simulink library "ObjSelect_lib"  (R2019b)
settings: Solver=VariableStepAuto  StartTime=0.0  StopTime=10.0  RelTol=1e-3
libraries: $bdroot x1
settings Model: Creator=liuyi  LastModifiedBy=86156
settings DataIOCC: ReturnWorkspaceOutputs=off
settings DebuggingCC: ArithmeticOperatorsInVariantConditions=warning
settings SFSimCC: SimUseLocalCustomCode=off  CustomCodeUndefinedFunction=UseInterfaceOnly
settings RTWCC: RTWUseLocalCustomCode=off
settings CodeAppCC: StateflowObjectComments=on

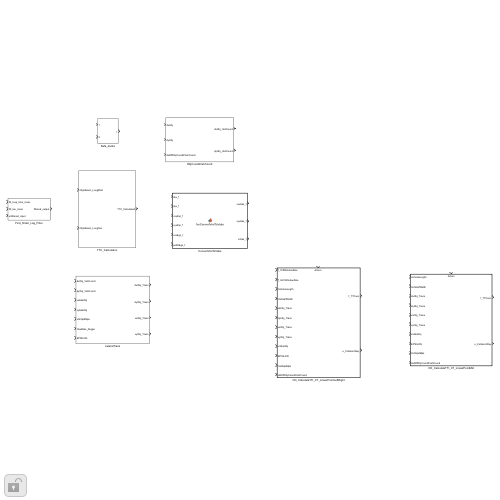
[thumbnail: Simulink's stored preview of the top-level diagram]
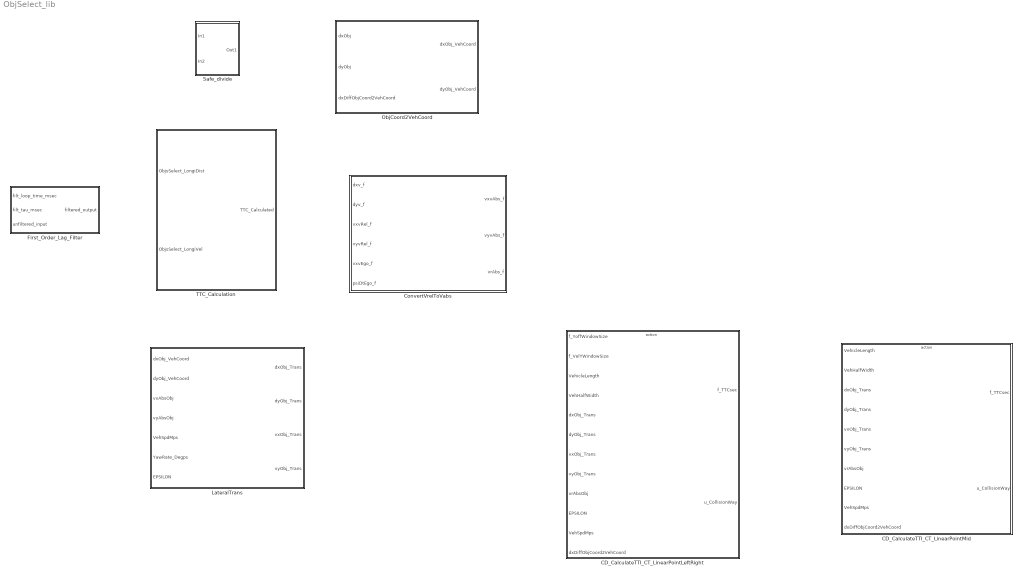
== system ObjSelect_lib ==
  CD_CalculateTTI_CT_LinearPointLeftRight : Subsystem  TreatAsAtomicUnit=on
  CD_CalculateTTI_CT_LinearPointMid : Subsystem  TreatAsAtomicUnit=on
  ConvertVrelToVabs : MATLAB Function  TreatAsAtomicUnit=on
  First_Order_Lag_Filter : Subsystem
  LateralTrans : Subsystem
  ObjCoord2VehCoord : Subsystem
  Safe_divide : Subsystem
  TTC_Calculation : Subsystem

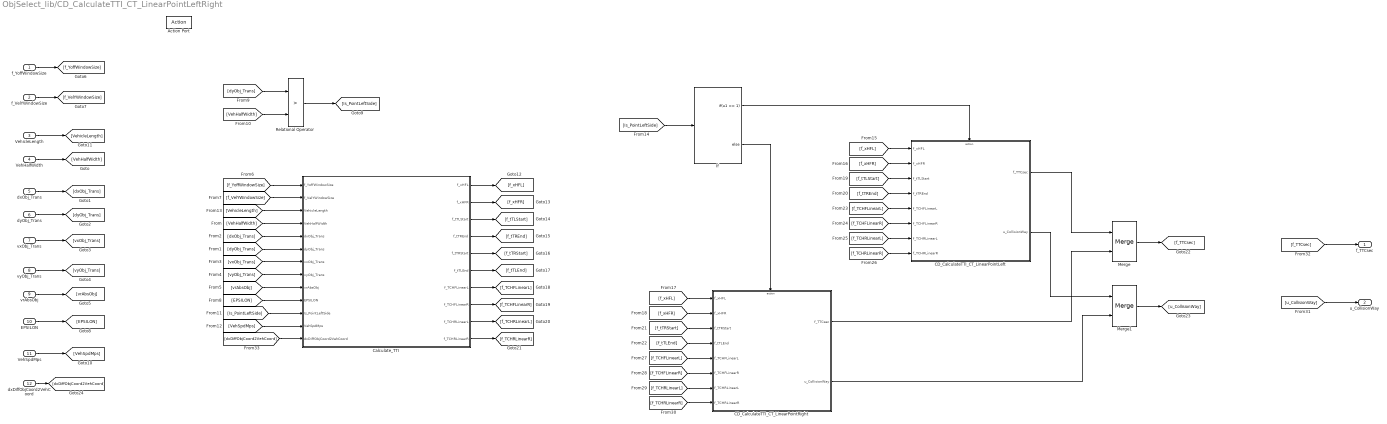
== system ObjSelect_lib/CD_CalculateTTI_CT_LinearPointLeftRight ==
  f_YoffWindowSize : Inport
  f_VelYWindowSize : Inport  Port=2
  VehicleLength : Inport  Port=3
  VehHalfWidth : Inport  Port=4
  dxObj_Trans : Inport  Port=5
  dyObj_Trans : Inport  Port=6
  vxObj_Trans : Inport  Port=7
  vyObj_Trans : Inport  Port=8
  vrAbsObj : Inport  Port=9
  EPSILON : Inport  Port=10
  VehSpdMps : Inport  Port=11
  dxDiffObjCoord2VehCoord : Inport  Port=12
  Action Port : ActionPort
  CD_CalculateTTI_CT_LinearPointLeft : Subsystem  TreatAsAtomicUnit=on
  "CD_CalculateTTI_CT_LinearPointRight " : Subsystem  TreatAsAtomicUnit=on
  Calculate_TTI : MATLAB Function  TreatAsAtomicUnit=on
  If : If  IfExpression=u1 == 1
  Merge : Merge
  Merge1 : Merge
  Relational Operator : RelationalOperator  Operator=>  OutDataTypeStr=boolean  RndMeth=Simplest
  f_TTCsec : Outport
  u_CollisionWay : Outport  Port=2
  wires:
  VehHalfWidth/1 -> [VehHalfWidth]
  dxObj_Trans/1 -> [dxObj_Trans]
  dyObj_Trans/1 -> [dyObj_Trans]
  vxObj_Trans/1 -> [vxObj_Trans]
  vyObj_Trans/1 -> [vyObj_Trans]
  vrAbsObj/1 -> [vrAbsObj]
  f_YoffWindowSize/1 -> [f_YoffWindowSize]
  f_VelYWindowSize/1 -> [f_VelYWindowSize]
  [f_YoffWindowSize] -> Calculate_TTI/1(f_YoffWindowSize)
  [f_VelYWindowSize] -> Calculate_TTI/2(f_VelYWindowSize)
  [VehHalfWidth] -> Calculate_TTI/4(VehHalfWidth)
  [dxObj_Trans] -> Calculate_TTI/5(dxObj_Trans)
  [dyObj_Trans] -> Calculate_TTI/6(dyObj_Trans)
  [vxObj_Trans] -> Calculate_TTI/7(vxObj_Trans)
  [vyObj_Trans] -> Calculate_TTI/8(vyObj_Trans)
  [vrAbsObj] -> Calculate_TTI/9(vrAbsObj)
  EPSILON/1 -> [EPSILON]
  [EPSILON] -> Calculate_TTI/10(EPSILON)
  [dyObj_Trans] -> Relational Operator/1
  [VehHalfWidth] -> Relational Operator/2
  Relational Operator/1 -> [Is_PointLeftSide]
  [Is_PointLeftSide] -> Calculate_TTI/11(Is_PointLeftSide)
  VehSpdMps/1 -> [VehSpdMps]
  [VehSpdMps] -> Calculate_TTI/12(VehSpdMps)
  VehicleLength/1 -> [VehicleLength]
  [VehicleLength] -> Calculate_TTI/3(VehicleLength)
  [Is_PointLeftSide] -> If/1
  If/1 -> CD_CalculateTTI_CT_LinearPointLeft/Action
  If/2 -> "CD_CalculateTTI_CT_LinearPointRight "/Action
  Calculate_TTI/1(f_xHFL) -> [f_xHFL]
  Calculate_TTI/2(f_xHFR) -> [f_xHFR]
  [f_xHFL] -> CD_CalculateTTI_CT_LinearPointLeft/1(f_xHFL)
  [f_xHFR] -> CD_CalculateTTI_CT_LinearPointLeft/2(f_xHFR)
  [f_xHFL] -> "CD_CalculateTTI_CT_LinearPointRight "/1(f_xHFL)
  [f_xHFR] -> "CD_CalculateTTI_CT_LinearPointRight "/2(f_xHFR)
  Calculate_TTI/3(f_tTLStart) -> [f_tTLStart]
  Calculate_TTI/4(f_tTREnd) -> [f_tTREnd]
  Calculate_TTI/5(f_tTRStart) -> [f_tTRStart]
  Calculate_TTI/6(f_tTLEnd) -> [f_tTLEnd]
  Calculate_TTI/7(f_TCHFLinearL) -> [f_TCHFLinearL]
  Calculate_TTI/8(f_TCHFLinearR) -> [f_TCHFLinearR]
  Calculate_TTI/9(f_TCHRLinearL) -> [f_TCHRLinearL]
  Calculate_TTI/10(f_TCHRLinearR) -> [f_TCHRLinearR]
  [f_tTLStart] -> CD_CalculateTTI_CT_LinearPointLeft/3(f_tTLStart)
  [f_tTREnd] -> CD_CalculateTTI_CT_LinearPointLeft/4(f_tTREnd)
  [f_TCHFLinearL] -> CD_CalculateTTI_CT_LinearPointLeft/5(f_TCHFLinearL)
  [f_TCHFLinearR] -> CD_CalculateTTI_CT_LinearPointLeft/6(f_TCHFLinearR)
  [f_TCHRLinearL] -> CD_CalculateTTI_CT_LinearPointLeft/7(f_TCHRLinearL)
  [f_TCHRLinearR] -> CD_CalculateTTI_CT_LinearPointLeft/8(f_TCHRLinearR)
  [f_tTRStart] -> "CD_CalculateTTI_CT_LinearPointRight "/3(f_tTRStart)
  [f_tTLEnd] -> "CD_CalculateTTI_CT_LinearPointRight "/4(f_tTLEnd)
  [f_TCHFLinearL] -> "CD_CalculateTTI_CT_LinearPointRight "/5(f_TCHFLinearL)
  [f_TCHFLinearR] -> "CD_CalculateTTI_CT_LinearPointRight "/6(f_TCHFLinearR)
  [f_TCHRLinearL] -> "CD_CalculateTTI_CT_LinearPointRight "/7(f_TCHRLinearL)
  [f_TCHRLinearR] -> "CD_CalculateTTI_CT_LinearPointRight "/8(f_TCHRLinearR)
  CD_CalculateTTI_CT_LinearPointLeft/1(f_TTCsec) -> Merge/1
  "CD_CalculateTTI_CT_LinearPointRight "/1(f_TTCsec) -> Merge/2
  CD_CalculateTTI_CT_LinearPointLeft/2(u_CollisionWay) -> Merge1/1
  "CD_CalculateTTI_CT_LinearPointRight "/2(u_CollisionWay) -> Merge1/2
  [f_TTCsec] -> f_TTCsec/1
  [u_CollisionWay] -> u_CollisionWay/1
  Merge/1 -> [f_TTCsec]
  Merge1/1 -> [u_CollisionWay]
  dxDiffObjCoord2VehCoord/1 -> [dxDiffObjCoord2VehCoord]
  [dxDiffObjCoord2VehCoord] -> Calculate_TTI/13(dxDiffObjCoord2VehCoord)

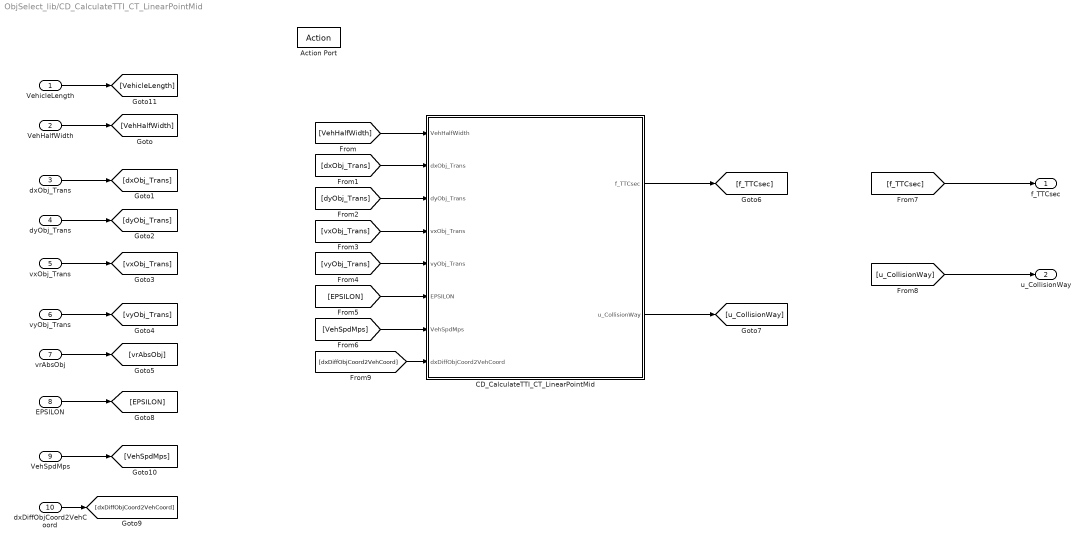
== system ObjSelect_lib/CD_CalculateTTI_CT_LinearPointMid ==
  VehicleLength : Inport
  VehHalfWidth : Inport  Port=2
  dxObj_Trans : Inport  Port=3
  dyObj_Trans : Inport  Port=4
  vxObj_Trans : Inport  Port=5
  vyObj_Trans : Inport  Port=6
  vrAbsObj : Inport  Port=7
  EPSILON : Inport  Port=8
  VehSpdMps : Inport  Port=9
  dxDiffObjCoord2VehCoord : Inport  Port=10
  Action Port : ActionPort
  CD_CalculateTTI_CT_LinearPointMid : MATLAB Function  TreatAsAtomicUnit=on
  f_TTCsec : Outport
  u_CollisionWay : Outport  Port=2  OutDataTypeStr=uint8
  wires:
  VehHalfWidth/1 -> [VehHalfWidth]
  dxObj_Trans/1 -> [dxObj_Trans]
  dyObj_Trans/1 -> [dyObj_Trans]
  vxObj_Trans/1 -> [vxObj_Trans]
  vyObj_Trans/1 -> [vyObj_Trans]
  vrAbsObj/1 -> [vrAbsObj]
  EPSILON/1 -> [EPSILON]
  VehSpdMps/1 -> [VehSpdMps]
  VehicleLength/1 -> [VehicleLength]
  [VehHalfWidth] -> CD_CalculateTTI_CT_LinearPointMid/1(VehHalfWidth)
  [dxObj_Trans] -> CD_CalculateTTI_CT_LinearPointMid/2(dxObj_Trans)
  [dyObj_Trans] -> CD_CalculateTTI_CT_LinearPointMid/3(dyObj_Trans)
  [vxObj_Trans] -> CD_CalculateTTI_CT_LinearPointMid/4(vxObj_Trans)
  [vyObj_Trans] -> CD_CalculateTTI_CT_LinearPointMid/5(vyObj_Trans)
  [EPSILON] -> CD_CalculateTTI_CT_LinearPointMid/6(EPSILON)
  [VehSpdMps] -> CD_CalculateTTI_CT_LinearPointMid/7(VehSpdMps)
  CD_CalculateTTI_CT_LinearPointMid/2(u_CollisionWay) -> [u_CollisionWay]
  [f_TTCsec] -> f_TTCsec/1
  [u_CollisionWay] -> u_CollisionWay/1
  CD_CalculateTTI_CT_LinearPointMid/1(f_TTCsec) -> [f_TTCsec]
  dxDiffObjCoord2VehCoord/1 -> [dxDiffObjCoord2VehCoord]
  [dxDiffObjCoord2VehCoord] -> CD_CalculateTTI_CT_LinearPointMid/8(dxDiffObjCoord2VehCoord)

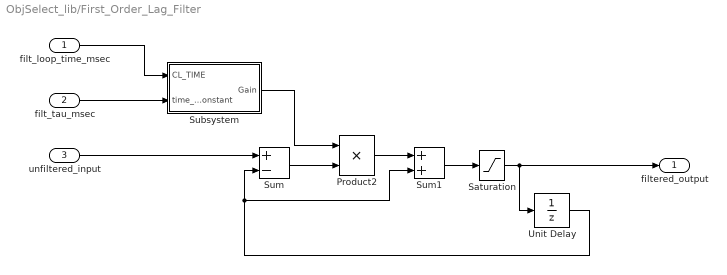
== system ObjSelect_lib/First_Order_Lag_Filter ==
  filt_loop_time_msec : Inport
  filt_tau_msec : Inport  Port=2
  unfiltered_input : Inport  Port=3
  Product2 : Product  Description=_GWMAB30P4.LKAFN.000_153_  Inputs=**  InputSameDT=on  OutDataTypeStr=Inherit: Same as first input
  Saturation : Saturate  Description=_GWMAB30P4.LKAFN.000_154_  UpperLimit=65535  LowerLimit=-65535
  Subsystem : Subsystem
  Sum : Sum  Description=_GWMAB30P4.LKAFN.000_155_  Inputs=+-  InputSameDT=on  OutDataTypeStr=Inherit: Same as first input
  Sum1 : Sum  Description=_GWMAB30P4.LKAFN.000_156_  InputSameDT=on  OutDataTypeStr=Inherit: Same as first input
  Unit Delay : UnitDelay  Description=_GWMAB30P4.LKAFN.000_157_  SampleTime=-1  HasFrameUpgradeWarning=on
  filtered_output : Outport
  wires:
  Unit Delay/1 -> Sum1/2, Sum/2
  Saturation/1 -> Unit Delay/1, filtered_output/1
  Product2/1 -> Sum1/1
  unfiltered_input/1 -> Sum/1
  Sum1/1 -> Saturation/1
  filt_tau_msec/1 -> Subsystem/2(time_constant)
  Sum/1 -> Product2/2
  filt_loop_time_msec/1 -> Subsystem/1(CL_TIME)
  Subsystem/1(Gain) -> Product2/1

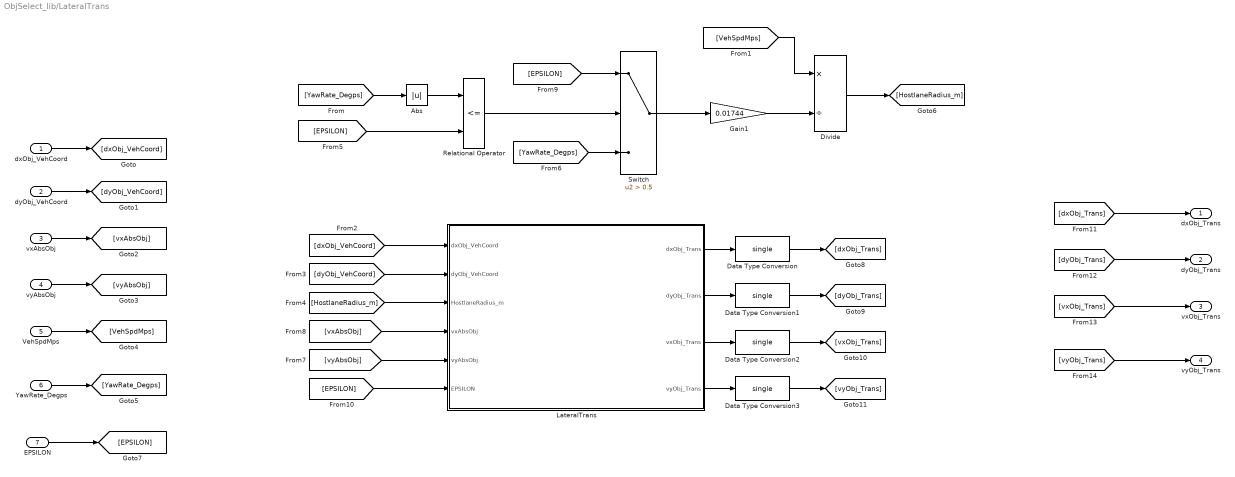
== system ObjSelect_lib/LateralTrans ==
  dxObj_VehCoord : Inport
  dyObj_VehCoord : Inport  Port=2
  vxAbsObj : Inport  Port=3
  vyAbsObj : Inport  Port=4
  VehSpdMps : Inport  Port=5
  YawRate_Degps : Inport  Port=6
  EPSILON : Inport  Port=7
  Abs : Abs
  Data Type Conversion{,1..3} (4 alike) : DataTypeConversion  OutDataTypeStr=single
  Divide : Product  Inputs=*/
  Gain1 : Gain  Gain=0.01744
  LateralTrans : MATLAB Function  TreatAsAtomicUnit=on
  Relational Operator : RelationalOperator  Operator=<=  OutDataTypeStr=boolean  RndMeth=Simplest
  Switch : Switch  Criteria=u2 > Threshold  Threshold=0.5
  dxObj_Trans : Outport
  dyObj_Trans : Outport  Port=2
  vxObj_Trans : Outport  Port=3
  vyObj_Trans : Outport  Port=4
  wires:
  dxObj_VehCoord/1 -> [dxObj_VehCoord]
  dyObj_VehCoord/1 -> [dyObj_VehCoord]
  vxAbsObj/1 -> [vxAbsObj]
  vyAbsObj/1 -> [vyAbsObj]
  VehSpdMps/1 -> [VehSpdMps]
  YawRate_Degps/1 -> [YawRate_Degps]
  [YawRate_Degps] -> Abs/1
  Abs/1 -> Relational Operator/1
  Gain1/1 -> Divide/2
  [VehSpdMps] -> Divide/1
  Divide/1 -> [HostlaneRadius_m]
  [dxObj_VehCoord] -> LateralTrans/1(dxObj_VehCoord)
  [dyObj_VehCoord] -> LateralTrans/2(dyObj_VehCoord)
  [HostlaneRadius_m] -> LateralTrans/3(HostlaneRadius_m)
  [vxAbsObj] -> LateralTrans/4(vxAbsObj)
  [vyAbsObj] -> LateralTrans/5(vyAbsObj)
  [EPSILON] -> Relational Operator/2
  Relational Operator/1 -> Switch/2
  [YawRate_Degps] -> Switch/3
  [EPSILON] -> Switch/1
  Switch/1 -> Gain1/1
  [EPSILON] -> LateralTrans/6(EPSILON)
  LateralTrans/1(dxObj_Trans) -> Data Type Conversion/1
  LateralTrans/2(dyObj_Trans) -> Data Type Conversion1/1
  LateralTrans/3(vxObj_Trans) -> Data Type Conversion2/1
  LateralTrans/4(vyObj_Trans) -> Data Type Conversion3/1
  [dxObj_Trans] -> dxObj_Trans/1
  [vxObj_Trans] -> vxObj_Trans/1
  [dyObj_Trans] -> dyObj_Trans/1
  [vyObj_Trans] -> vyObj_Trans/1
  EPSILON/1 -> [EPSILON]
  Data Type Conversion/1 -> [dxObj_Trans]
  Data Type Conversion1/1 -> [dyObj_Trans]
  Data Type Conversion2/1 -> [vxObj_Trans]
  Data Type Conversion3/1 -> [vyObj_Trans]

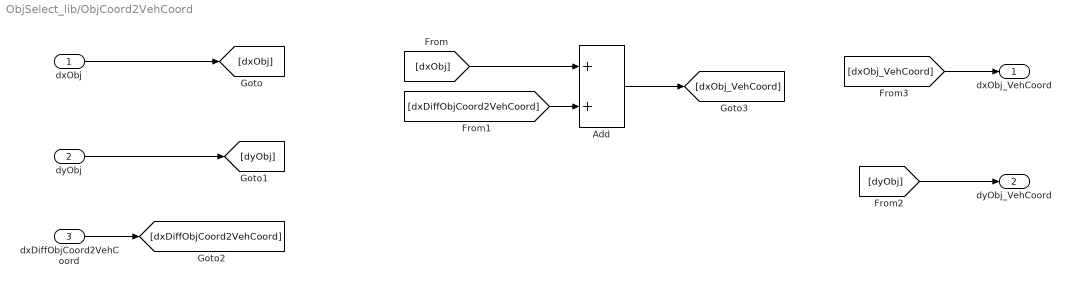
== system ObjSelect_lib/ObjCoord2VehCoord ==
  dxObj : Inport
  dyObj : Inport  Port=2
  dxDiffObjCoord2VehCoord : Inport  Port=3
  Add : Sum
  dxObj_VehCoord : Outport
  dyObj_VehCoord : Outport  Port=2
  wires:
  dxObj/1 -> [dxObj]
  dyObj/1 -> [dyObj]
  dxDiffObjCoord2VehCoord/1 -> [dxDiffObjCoord2VehCoord]
  [dxObj] -> Add/1
  [dxDiffObjCoord2VehCoord] -> Add/2
  [dyObj] -> dyObj_VehCoord/1
  Add/1 -> [dxObj_VehCoord]
  [dxObj_VehCoord] -> dxObj_VehCoord/1

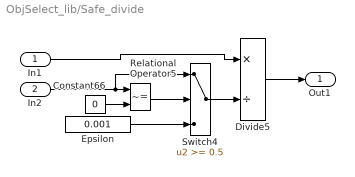
== system ObjSelect_lib/Safe_divide ==
  In1 : Inport
  In2 : Inport  Port=2
  Constant66 : Constant  Description=_GWMH9P3.LKAFN.000_31_  Value=0
  Divide5 : Product  Description=_GWMH9P3.LKAFN.000_32_  Inputs=*/
  Epsilon : Constant  Description=_GWMH9P3.LKAFN.000_33_  Value=0.001
  Relational Operator5 : RelationalOperator  Description=_GWMH9P3.LKAFN.000_34_  Operator=~=  OutDataTypeStr=boolean  RndMeth=Nearest
  Switch4 : Switch  Description=_GWMH9P3.LKAFN.000_35_  Threshold=0.5  OutDataTypeStr=Inherit: Inherit via back propagation
  Out1 : Outport
  wires:
  In2/1 -> Switch4/1, Relational Operator5/1
  In1/1 -> Divide5/1
  Relational Operator5/1 -> Switch4/2
  Divide5/1 -> Out1/1
  Constant66/1 -> Relational Operator5/2
  Switch4/1 -> Divide5/2
  Epsilon/1 -> Switch4/3

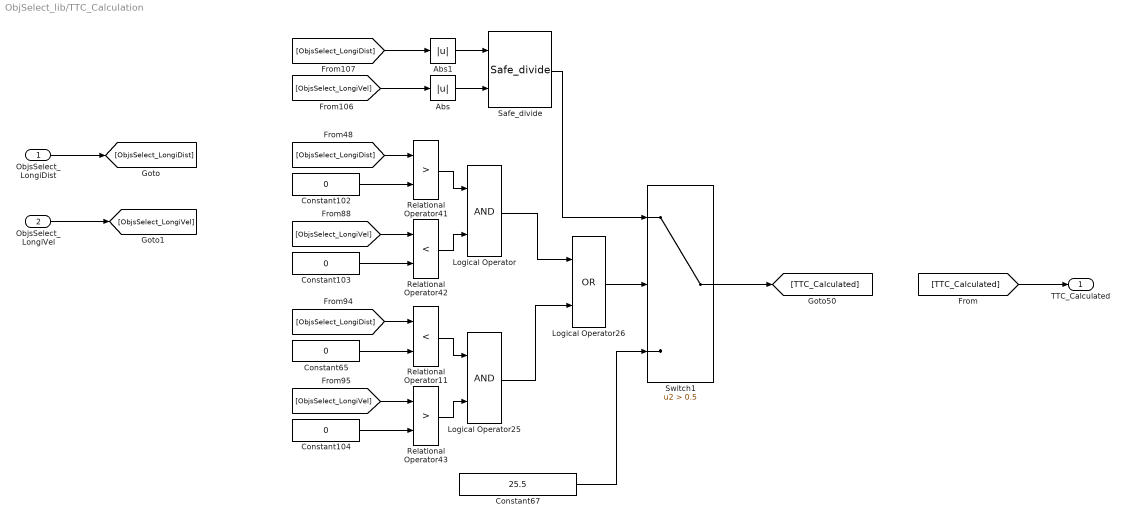
== system ObjSelect_lib/TTC_Calculation ==
  ObjsSelect_LongiDist : Inport
  ObjsSelect_LongiVel : Inport  Port=2
  Abs : Abs
  Abs1 : Abs
  Constant{65,102..104} (4 alike) : Constant  Description=_GWMH9P5.ELK.000_37_  Value=0
  Constant67 : Constant  Description=_GWMH9P5.ELK.000_38_  Value=25.5  OutDataTypeStr=single
  Logical Operator : Logic  AllPortsSameDT=off  OutDataTypeStr=boolean
  Logical Operator25 : Logic  AllPortsSameDT=off  OutDataTypeStr=boolean
  Logical Operator26 : Logic  Operator=OR  AllPortsSameDT=off  OutDataTypeStr=boolean
  Relational Operator11 : RelationalOperator  Description=_GWMH9P5.ELK.000_104_  Operator=<  OutDataTypeStr=boolean  RndMeth=Nearest
  Relational Operator41 : RelationalOperator  Description=_GWMH9P5.ELK.000_104_  Operator=>  OutDataTypeStr=boolean  RndMeth=Nearest
  Relational Operator42 : RelationalOperator  Description=_GWMH9P5.ELK.000_104_  Operator=<  OutDataTypeStr=boolean  RndMeth=Nearest
  Relational Operator43 : RelationalOperator  Description=_GWMH9P5.ELK.000_104_  Operator=>  OutDataTypeStr=boolean  RndMeth=Nearest
  Safe_divide : $bdroot/Safe_divide  SystemSampleTime=-1  Latency=0  AutoFrameSizeCalculation=off
  Switch1 : Switch  Description=_GWMH9P5.ELK.000_119_  Criteria=u2 > Threshold  Threshold=0.5  OutDataTypeStr=single
  TTC_Calculated : Outport
  wires:
  [ObjsSelect_LongiDist] -> Abs1/1
  Logical Operator25/1 -> Logical Operator26/2
  Constant65/1 -> Relational Operator11/2
  Abs/1 -> Safe_divide/2
  [ObjsSelect_LongiVel] -> Abs/1
  [ObjsSelect_LongiVel] -> Relational Operator42/1
  Logical Operator26/1 -> Switch1/2
  [ObjsSelect_LongiVel] -> Relational Operator43/1
  Constant104/1 -> Relational Operator43/2
  Constant103/1 -> Relational Operator42/2
  Relational Operator11/1 -> Logical Operator25/1
  Abs1/1 -> Safe_divide/1
  Logical Operator/1 -> Logical Operator26/1
  Relational Operator42/1 -> Logical Operator/2
  Relational Operator43/1 -> Logical Operator25/2
  Constant102/1 -> Relational Operator41/2
  [ObjsSelect_LongiDist] -> Relational Operator41/1
  Constant67/1 -> Switch1/3
  Switch1/1 -> [TTC_Calculated]
  Safe_divide/1 -> Switch1/1
  Relational Operator41/1 -> Logical Operator/1
  [ObjsSelect_LongiDist] -> Relational Operator11/1
  [TTC_Calculated] -> TTC_Calculated/1
  ObjsSelect_LongiDist/1 -> [ObjsSelect_LongiDist]
  ObjsSelect_LongiVel/1 -> [ObjsSelect_LongiVel]

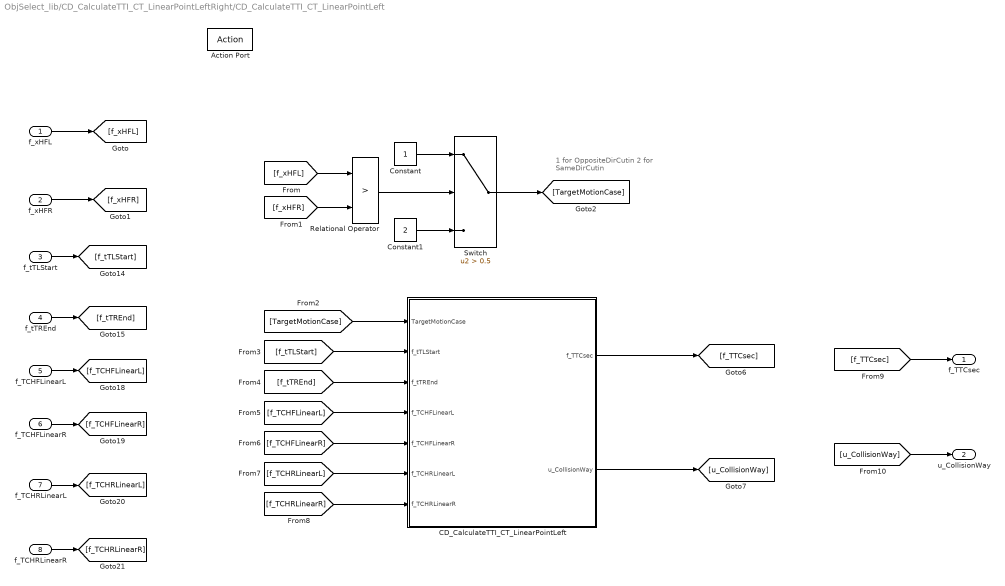
== system ObjSelect_lib/CD_CalculateTTI_CT_LinearPointLeftRight/CD_CalculateTTI_CT_LinearPointLeft ==
  note: 1 for OppositeDirCutin
      | 2 for SameDirCutin
  f_xHFL : Inport
  f_xHFR : Inport  Port=2
  f_tTLStart : Inport  Port=3
  f_tTREnd : Inport  Port=4
  f_TCHFLinearL : Inport  Port=5
  f_TCHFLinearR : Inport  Port=6
  f_TCHRLinearL : Inport  Port=7
  f_TCHRLinearR : Inport  Port=8
  Action Port : ActionPort
  CD_CalculateTTI_CT_LinearPointLeft : MATLAB Function  TreatAsAtomicUnit=on
  Constant : Constant
  Constant1 : Constant  Value=2
  Relational Operator : RelationalOperator  Operator=>  OutDataTypeStr=boolean  RndMeth=Simplest
  Switch : Switch  Criteria=u2 > Threshold  Threshold=0.5
  f_TTCsec : Outport
  u_CollisionWay : Outport  Port=2  OutDataTypeStr=uint8
  wires:
  f_xHFL/1 -> [f_xHFL]
  f_xHFR/1 -> [f_xHFR]
  [f_xHFL] -> Relational Operator/1
  [f_xHFR] -> Relational Operator/2
  Relational Operator/1 -> Switch/2
  Constant/1 -> Switch/1
  Constant1/1 -> Switch/3
  Switch/1 -> [TargetMotionCase]
  [TargetMotionCase] -> CD_CalculateTTI_CT_LinearPointLeft/1(TargetMotionCase)
  f_tTLStart/1 -> [f_tTLStart]
  f_tTREnd/1 -> [f_tTREnd]
  f_TCHFLinearL/1 -> [f_TCHFLinearL]
  f_TCHFLinearR/1 -> [f_TCHFLinearR]
  f_TCHRLinearR/1 -> [f_TCHRLinearR]
  f_TCHRLinearL/1 -> [f_TCHRLinearL]
  [f_tTLStart] -> CD_CalculateTTI_CT_LinearPointLeft/2(f_tTLStart)
  [f_tTREnd] -> CD_CalculateTTI_CT_LinearPointLeft/3(f_tTREnd)
  [f_TCHFLinearL] -> CD_CalculateTTI_CT_LinearPointLeft/4(f_TCHFLinearL)
  [f_TCHFLinearR] -> CD_CalculateTTI_CT_LinearPointLeft/5(f_TCHFLinearR)
  [f_TCHRLinearL] -> CD_CalculateTTI_CT_LinearPointLeft/6(f_TCHRLinearL)
  [f_TCHRLinearR] -> CD_CalculateTTI_CT_LinearPointLeft/7(f_TCHRLinearR)
  CD_CalculateTTI_CT_LinearPointLeft/2(u_CollisionWay) -> [u_CollisionWay]
  [f_TTCsec] -> f_TTCsec/1
  [u_CollisionWay] -> u_CollisionWay/1
  CD_CalculateTTI_CT_LinearPointLeft/1(f_TTCsec) -> [f_TTCsec]

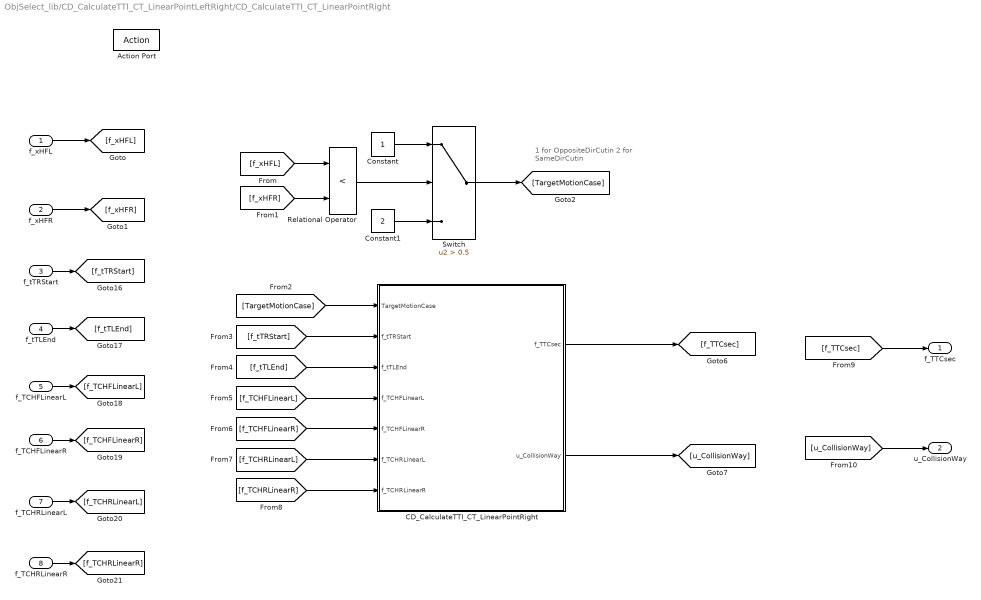
== system ObjSelect_lib/CD_CalculateTTI_CT_LinearPointLeftRight/CD_CalculateTTI_CT_LinearPointRight  ==
  note: 1 for OppositeDirCutin
      | 2 for SameDirCutin
  f_xHFL : Inport
  f_xHFR : Inport  Port=2
  f_tTRStart : Inport  Port=3
  f_tTLEnd : Inport  Port=4
  f_TCHFLinearL : Inport  Port=5
  f_TCHFLinearR : Inport  Port=6
  f_TCHRLinearL : Inport  Port=7
  f_TCHRLinearR : Inport  Port=8
  Action Port : ActionPort
  CD_CalculateTTI_CT_LinearPointRight : MATLAB Function  TreatAsAtomicUnit=on
  Constant : Constant
  Constant1 : Constant  Value=2
  Relational Operator : RelationalOperator  Operator=<  OutDataTypeStr=boolean  RndMeth=Simplest
  Switch : Switch  Criteria=u2 > Threshold  Threshold=0.5
  f_TTCsec : Outport
  u_CollisionWay : Outport  Port=2  OutDataTypeStr=uint8
  wires:
  [f_xHFL] -> Relational Operator/1
  [f_xHFR] -> Relational Operator/2
  Relational Operator/1 -> Switch/2
  Constant/1 -> Switch/1
  Constant1/1 -> Switch/3
  Switch/1 -> [TargetMotionCase]
  f_xHFL/1 -> [f_xHFL]
  f_xHFR/1 -> [f_xHFR]
  f_tTRStart/1 -> [f_tTRStart]
  f_tTLEnd/1 -> [f_tTLEnd]
  f_TCHFLinearL/1 -> [f_TCHFLinearL]
  f_TCHFLinearR/1 -> [f_TCHFLinearR]
  f_TCHRLinearL/1 -> [f_TCHRLinearL]
  f_TCHRLinearR/1 -> [f_TCHRLinearR]
  [TargetMotionCase] -> CD_CalculateTTI_CT_LinearPointRight/1(TargetMotionCase)
  [f_tTRStart] -> CD_CalculateTTI_CT_LinearPointRight/2(f_tTRStart)
  [f_tTLEnd] -> CD_CalculateTTI_CT_LinearPointRight/3(f_tTLEnd)
  [f_TCHFLinearL] -> CD_CalculateTTI_CT_LinearPointRight/4(f_TCHFLinearL)
  [f_TCHFLinearR] -> CD_CalculateTTI_CT_LinearPointRight/5(f_TCHFLinearR)
  [f_TCHRLinearL] -> CD_CalculateTTI_CT_LinearPointRight/6(f_TCHRLinearL)
  [f_TCHRLinearR] -> CD_CalculateTTI_CT_LinearPointRight/7(f_TCHRLinearR)
  CD_CalculateTTI_CT_LinearPointRight/2(u_CollisionWay) -> [u_CollisionWay]
  [f_TTCsec] -> f_TTCsec/1
  [u_CollisionWay] -> u_CollisionWay/1
  CD_CalculateTTI_CT_LinearPointRight/1(f_TTCsec) -> [f_TTCsec]

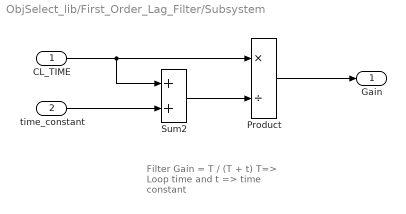
== system ObjSelect_lib/First_Order_Lag_Filter/Subsystem ==
  note: Filter Gain = T / (T + t)
      | T=> Loop time and
      | t => time constant
  CL_TIME : Inport
  time_constant : Inport  Port=2
  Product : Product  Description=_GWMAB30P4.LKAFN.000_144_  Inputs=*/  InputSameDT=on  OutDataTypeStr=Inherit: Same as first input
  Sum2 : Sum  Description=_GWMAB30P4.LKAFN.000_145_  InputSameDT=on  OutDataTypeStr=Inherit: Same as first input
  Gain : Outport
  wires:
  Sum2/1 -> Product/2
  Product/1 -> Gain/1
  CL_TIME/1 -> Product/1, Sum2/1
  time_constant/1 -> Sum2/2

== matlab function ObjSelect_lib/LateralTrans/LateralTrans ==
  data: dxObj_VehCoord input; dxObj_Trans output; dyObj_VehCoord input; HostlaneRadius_m input; vxAbsObj input; vyAbsObj input; EPSILON input; dyObj_Trans output; vxObj_Trans output; vyObj_Trans output
function [dxObj_Trans,dyObj_Trans,vxObj_Trans,vyObj_Trans] = fcn(dxObj_VehCoord,dyObj_VehCoord,HostlaneRadius_m,vxAbsObj,vyAbsObj,EPSILON)

f_TarXin = dxObj_VehCoord;
f_TarYin = dyObj_VehCoord;
f_TarVelXin = vxAbsObj;
f_TarVelYin = vyAbsObj;
f_HostlaneRadius_m = HostlaneRadius_m;

f_roTarget = sqrt((f_TarXin * f_TarXin) + (f_HostlaneRadius_m-f_TarYin) * (f_HostlaneRadius_m-f_TarYin));

%% Right turn
if (f_HostlaneRadius_m <= 0)
    if (f_roTarget < EPSILON)
        f_roTarget = EPSILON;
    end
    f_sinCta = f_TarXin/f_roTarget;
    f_targetRadiusCta = asin(f_sinCta);
    f_cosCta = sqrt(1-f_sinCta*f_sinCta);
    %% left side of straight
    if (f_roTarget > -f_HostlaneRadius_m)
        %%PointStraight_posX = f_roTarget * f_targetRadiusCta;
        PointStraight_posX = (-f_HostlaneRadius_m) * f_targetRadiusCta;
        PointStraight_posY = f_roTarget + f_HostlaneRadius_m;

        PointStraight_velX = (f_TarVelXin * f_cosCta) - (f_TarVelYin*f_sinCta);
        PointStraight_velY = (f_TarVelYin * f_cosCta) + (f_TarVelXin *f_sinCta);
    %% right side of straight
    else
        PointStraight_posX = (-f_HostlaneRadius_m * f_targetRadiusCta);
        PointStraight_posY = f_roTarget + f_HostlaneRadius_m;

        PointStraight_velX = (f_TarVelXin * f_cosCta) - (f_TarVelYin*f_sinCta);
        PointStraight_velY = (f_TarVelYin * f_cosCta) + (f_TarVelXin *f_sinCta);
    end
%% Left turn
else
    %% case out side and inside, start with --  inside --  left side of straight
    if(abs(f_HostlaneRadius_m - f_TarYin) < EPSILON)
        f_HostlaneRadius_m =  f_TarYin + (3.0*EPSILON);
    end
    f_targetRadiusCta = atan(f_TarXin/(f_HostlaneRadius_m - f_TarYin));
    f_sinCta = sin(f_targetRadiusCta);
    f_cosCta = cos(f_targetRadiusCta);
    %% left side of straight
    if (f_roTarget < f_HostlaneRadius_m)
        PointStraight_posX = f_HostlaneRadius_m * f_targetRadiusCta;
        PointStraight_posY = f_HostlaneRadius_m - f_roTarget;

        PointStraight_velX = (f_TarVelYin * f_sinCta) + (f_TarVelXin * f_cosCta);
        PointStraight_velY = (-f_TarVelXin * f_sinCta) + (f_TarVelYin * f_cosCta);
    %% right side of straight
    else
        PointStraight_posX = (f_HostlaneRadius_m * f_targetRadiusCta);
        PointStraight_posY = f_HostlaneRadius_m - f_roTarget;

        PointStraight_velX = (f_TarVelYin * f_sinCta) + (f_TarVelXin * f_cosCta);
        PointStraight_velY = (-f_TarVelXin * f_sinCta) + (f_TarVelYin * f_cosCta);
    end
end

dxObj_Trans = PointStraight_posX;
dyObj_Trans = PointStraight_posY;
vxObj_Trans = PointStraight_velX;
vyObj_Trans = PointStraight_velY;

== matlab function ObjSelect_lib/ConvertVrelToVabs ==
  data: dxv_f input; vxvAbs_f output; dyv_f input; vxvRel_f input; vyvRel_f input; vxvEgo_f input; psiDtEgo_f input; vyvAbs_f output; vrAbs_f output
function [vxvAbs_f, vyvAbs_f, vrAbs_f] = fcnConvertVrelToVabs(dxv_f, dyv_f, vxvRel_f, vyvRel_f, vxvEgo_f, psiDtEgo_f)

if (dxv_f ~= 0)
   t_radObjAngleToRear_f = atan(dyv_f / dxv_f);
else
   t_radObjAngleToRear_f = single(0.0);
end

t_dvRadial_f = sqrt(dxv_f * dxv_f + dyv_f * dyv_f);

t_vvRadial_f = t_dvRadial_f * psiDtEgo_f;

t_sinObjAngle_f = sin(t_radObjAngleToRear_f);
t_cosObjAngle_f = cos(t_radObjAngleToRear_f);

t_tempvx_f = (vxvRel_f * t_cosObjAngle_f) + vyvRel_f * t_sinObjAngle_f;
t_tempvy_f = (vxvRel_f * (-t_sinObjAngle_f)) + vyvRel_f * t_cosObjAngle_f;

t_tempvy_f = t_tempvy_f + t_vvRadial_f;

vxvAbs_f = ((t_tempvx_f * t_cosObjAngle_f) - (t_tempvy_f * t_sinObjAngle_f)) + vxvEgo_f;
vyvAbs_f = (t_tempvx_f * t_sinObjAngle_f) + (t_tempvy_f * t_cosObjAngle_f);
vrAbs_f = sqrt(vxvAbs_f * vxvAbs_f + vyvAbs_f * vyvAbs_f);

== matlab function ObjSelect_lib/CD_CalculateTTI_CT_LinearPointLeftRight/CD_CalculateTTI_CT_LinearPointLeft/CD_CalculateTTI_CT_LinearPointLeft ==
  data: TargetMotionCase input; f_TTCsec output; f_tTLStart input; f_tTREnd input; f_TCHFLinearL input; f_TCHFLinearR input; f_TCHRLinearL input; f_TCHRLinearR input; u_CollisionWay output
function [f_TTCsec,u_CollisionWay] = fcn(TargetMotionCase,f_tTLStart,f_tTREnd,f_TCHFLinearL,f_TCHFLinearR,f_TCHRLinearL,f_TCHRLinearR)

f_THFrLe = f_TCHFLinearL;
f_THFrRi = f_TCHFLinearR;
f_THReLe = f_TCHRLinearL;
f_THReRi = f_TCHRLinearR;

f_TTCsec = single(25.5);
u_CollisionWay = uint8(0); %% no collision

switch (TargetMotionCase)
    case 2 %% SameDirCutin
        if ( (f_tTLStart > f_THReRi) && (f_THReRi > 0.0) )
            f_TTCsec = single(25.5);
           u_CollisionWay = uint8(2); %% no collision target pass rear
        elseif ( (f_THFrLe > f_tTREnd) && (f_tTREnd > 0.0) )
            f_TTCsec = single(25.5);
            u_CollisionWay = uint8(6); %% no collision target pass front
        elseif ( (f_tTLStart > f_THReLe) && (f_THReLe > 0.0) && (f_tTREnd > f_THReRi) && (f_THReRi > 0.0) )
            f_TTCsec = single(25.5);
            u_CollisionWay = uint8(3); %% no collision, close, target following Host rear
        elseif ( (f_tTLStart > f_THFrLe) && (f_THFrLe > 0.0) && (f_tTLStart < f_THReLe) && (f_tTLStart > 0.0) )
            f_TTCsec = f_tTLStart;
            u_CollisionWay = uint8(1); %% target hit host at left side
        elseif ( (f_tTLStart <= f_THFrLe) && (f_tTLStart > 0.0) && (f_tTREnd > f_THFrRi) && (f_THFrRi > 0.0) )
            f_TTCsec = 0.5*(f_THFrLe + f_THFrRi);  %% @todo  refine according the  which side far from host moving direction/ current position
            u_CollisionWay = uint8(7); %% host hit target at front in lane
        elseif ( (f_tTLStart < f_THFrLe) && (f_tTLStart > 0.0) && (f_tTREnd < f_THFrRi) && (f_tTREnd > 0.0) )
            f_TTCsec = 0.5*(f_tTLStart + f_tTREnd);
            u_CollisionWay = uint8(8); %% no collision cut in    target pass host front
        elseif ( (f_tTLStart > f_THReLe) && (f_THReLe > 0.0) && (f_tTREnd < f_THReRi) && (f_tTREnd > 0.0) )
            f_TTCsec = 0.5*(f_tTLStart + f_tTREnd);
            u_CollisionWay = uint8(9); %% target hit host at rear
        else
            f_TTCsec = single(25.5);
            u_CollisionWay = uint8(4); %% @todo  other warning situation
        end
    case 1 %% OppositeDirCutin
        if ( (f_THReLe < f_tTLStart) && (f_THReLe > 0.0) )
            f_TTCsec = single(25.5);
            u_CollisionWay = uint8(12); %% no collision target pass rear
        elseif ( (f_tTREnd < f_THFrRi) )
            f_TTCsec = single(25.5);
            u_CollisionWay = uint8(16); %% no collision target pass front
        elseif ( (f_tTLStart > f_THFrLe) && (f_THFrLe > 0.0) && (f_tTLStart < f_THReLe) && (f_tTLStart > 0.0) )
            f_TTCsec = f_tTLStart;
            u_CollisionWay = uint8(11); %% target hit host at left side
        elseif ( (f_tTLStart <= f_THFrLe) && (f_tTLStart > 0.0) && (f_tTREnd > f_THFrRi) && (f_THFrRi > 0.0) )
            f_TTCsec = 0.5*(f_THFrLe + f_THFrRi); %% @todo  refine according the  which side far from host moving direction/ current position
			u_CollisionWay = uint8(17); %% host hit target at front in lane
        else
            f_TTCsec = single(25.5);
            u_CollisionWay = uint8(14); %% @todo  almost hit or other  situation
        end
end

== matlab function ObjSelect_lib/CD_CalculateTTI_CT_LinearPointLeftRight/CD_CalculateTTI_CT_LinearPointRight /CD_CalculateTTI_CT_LinearPointRight ==
  data: TargetMotionCase input; f_TTCsec output; f_tTRStart input; f_tTLEnd input; f_TCHFLinearL input; f_TCHFLinearR input; f_TCHRLinearL input; f_TCHRLinearR input; u_CollisionWay output
function [f_TTCsec,u_CollisionWay] = fcn(TargetMotionCase,f_tTRStart,f_tTLEnd,f_TCHFLinearL,f_TCHFLinearR,f_TCHRLinearL,f_TCHRLinearR)

f_THFrLe = f_TCHFLinearL;
f_THFrRi = f_TCHFLinearR;
f_THReLe = f_TCHRLinearL;
f_THReRi = f_TCHRLinearR;

f_TTCsec = single(25.5);
u_CollisionWay = uint8(0); %%no collision

switch (TargetMotionCase)
    case 2 %% SameDirCutin
        if ( (f_THFrRi > f_tTLEnd) && (f_tTLEnd > 0.0) )
            f_TTCsec = single(25.5);
            u_CollisionWay = uint8(26); %% no collision target pass front
        elseif ( (f_tTRStart > f_THReLe) && (f_THReLe > 0.0) )
            f_TTCsec = single(25.5);
            u_CollisionWay = uint8(22); %% no collision  target pass rear
        elseif ( ((f_tTRStart >= f_THReRi) && (f_THReRi > 0.0) && (f_tTLEnd <= f_THReLe) && (f_tTLEnd > 0.0)) )
            f_TTCsec = single(25.5);
            u_CollisionWay = uint8(29); %% target hit host at rear
        elseif ( (f_tTRStart >= f_THFrRi) && (f_THFrRi > 0.0) && (f_tTRStart <= f_THReRi) && (f_tTRStart > 0.0) )
            f_TTCsec = f_tTRStart;
            u_CollisionWay = uint8(21); %% target hit host at Right side
        elseif ( (f_tTLEnd >= f_THFrLe) && (f_THFrLe > 0.0) && (f_tTRStart <= f_THFrRi) && (f_tTRStart > 0.0) )
            f_TTCsec = 0.5*(f_THFrLe + f_THFrRi); %% @todo  refine according  which side far from host moving direction/ current position*/
            u_CollisionWay = uint8(27); %% host hit target at front
        elseif ( (f_tTLEnd < f_THFrLe) && (f_tTLEnd > 0.0) && (f_tTRStart < f_THFrRi) && (f_tTRStart > 0.0) )
            f_TTCsec = single(25.5);
            u_CollisionWay = uint8(28); %% cut in
        else
            f_TTCsec = single(25.5);
            u_CollisionWay = uint8(24); %% @todo  other warning situation
        end
    case 1 %% OppositeDirCutin
        if ( (f_THReRi < f_tTRStart) && (f_THReRi > 0.0) )
            f_TTCsec = single(25.5);
            u_CollisionWay = uint8(32); %% no collision target pass rear
        elseif ( (f_tTLEnd < f_THFrLe) && (f_tTLEnd > 0.0) )
            f_TTCsec = single(25.5);
            u_CollisionWay = uint8(36); %% no collision  target pass front
        elseif ( (f_tTRStart > f_THFrRi) && (f_THFrRi > 0.0) && (f_tTRStart < f_THReRi) && (f_tTRStart > 0.0) )
            f_TTCsec = f_tTRStart;
            u_CollisionWay = uint8(31); %% target hit host at Right side
        elseif ( (f_tTRStart <= f_THFrRi) && (f_tTRStart > 0.0) && (f_tTLEnd > f_THFrLe) && (f_THFrLe > 0.0) )
            f_TTCsec = 0.5*(f_THFrLe + f_THFrRi);  %% @todo  refine according which side far from host moving direction/ current position*/
            u_CollisionWay = uint8(37); %% host hit target at front
        else
            f_TTCsec = single(25.5);
            u_CollisionWay = uint8(34); %% @todo  almost hit or other  situation
        end
end

== matlab function ObjSelect_lib/CD_CalculateTTI_CT_LinearPointLeftRight/Calculate_TTI ==
  data: f_YoffWindowSize input; f_xHFL output; f_VelYWindowSize input; VehicleLength input; VehHalfWidth input; dxObj_Trans input; dyObj_Trans input; vxObj_Trans input; vyObj_Trans input; vrAbsObj input; EPSILON input; Is_PointLeftSide input; VehSpdMps input; f_xHFR output; f_tTLStart output; f_tTREnd output; f_tTRStart output; f_tTLEnd output; f_TCHFLinearL output; f_TCHFLinearR output; f_TCHRLinearL output; f_TCHRLinearR output; dxDiffObjCoord2VehCoord input
function [f_xHFL,f_xHFR,f_tTLStart,f_tTREnd,f_tTRStart,f_tTLEnd,f_TCHFLinearL,f_TCHFLinearR,f_TCHRLinearL,f_TCHRLinearR] = fcn(f_YoffWindowSize,f_VelYWindowSize,VehicleLength,VehHalfWidth,dxObj_Trans,dyObj_Trans,vxObj_Trans,vyObj_Trans,vrAbsObj,EPSILON,Is_PointLeftSide,VehSpdMps,dxDiffObjCoord2VehCoord)

f_VehLength = VehicleLength;
f_VehHalfWidth = VehHalfWidth;
f_TarX = dxObj_Trans;
f_TarY = dyObj_Trans;
f_TarVelX = vxObj_Trans;
f_TarVelY = vyObj_Trans;
f_TarVelr = vrAbsObj;
f_HostVrel = VehSpdMps;

f_xHFL = single(0.0);
f_xHFR = single(0.0);
f_tTLStart = single(0.0);
f_tTREnd = single(0.0);
f_tTRStart = single(0.0);
f_tTLEnd = single(0.0);
f_TCHFLinearL = single(0.0);
f_TCHFLinearR = single(0.0);
f_TCHRLinearL = single(0.0);
f_TCHRLinearR = single(0.0);

%% check the need to do CD calculation
if ( ((f_TarY > f_YoffWindowSize) && (f_TarVelY > f_VelYWindowSize)) || ((f_TarY < -f_YoffWindowSize) && (f_TarVelY < -f_VelYWindowSize)) )
    %% no collision expected -> TTI to DEFAULT
    f_tTLStart = single(0.0);
    f_tTREnd = single(0.0);
    f_tTRStart = single(0.0);
    f_tTLEnd = single(0.0);
    f_TCHFLinearL = single(0.0);
    f_TCHFLinearR = single(0.0);
    f_TCHRLinearL = single(0.0);
    f_TCHRLinearR = single(0.0);
else
    if (abs(f_TarVelY) > EPSILON)
        f_TarVslop = f_TarVelX / abs(f_TarVelY);
    else %% @todo   large slop, in case over flow
        f_TarVslop = 1000.0*f_TarVelX;
    end
    
    %% f_TarXYoff = f_TarX - f_TarY*f_TarVslop;
    %% two straight line collision cross X position for Host Front
    if (Is_PointLeftSide > 0.5) %%left side
        %%f_xHFL = (f_TarX + (f_TarVslop * (f_TarY - f_VehHalfWidth)));
        %%f_xHFR = (f_TarX + (f_TarVslop * (f_VehHalfWidth + f_TarY)));
        f_xHFL = (f_TarX + (f_TarVslop * (f_TarY - f_VehHalfWidth)) - dxDiffObjCoord2VehCoord);
        f_xHFR = (f_TarX + (f_TarVslop * (f_VehHalfWidth + f_TarY)) - dxDiffObjCoord2VehCoord);
    else %%right side
        %%f_xHFL = (f_TarX + (f_TarVslop * (f_VehHalfWidth - f_TarY)));
        %%f_xHFR = (f_TarX - (f_TarVslop * (f_VehHalfWidth + f_TarY)));
        f_xHFL = (f_TarX + (f_TarVslop * (f_VehHalfWidth - f_TarY)) - dxDiffObjCoord2VehCoord);
        f_xHFR = (f_TarX - (f_TarVslop * (f_VehHalfWidth + f_TarY)) - dxDiffObjCoord2VehCoord);
    end
    
    if (abs(f_TarVelr) < EPSILON)
        f_TarVelr = EPSILON;
    end
    
    %% f_inverseTvrr = FCN_Inv(f_TarVelr);
    %% Target to host trajectory time
    %%f_TtL = sqrt( ((f_VehHalfWidth - f_TarY)*(f_VehHalfWidth - f_TarY)) + ((f_TarX - f_xHFL)*(f_TarX - f_xHFL)) ) / (f_TarVelr);
    %%f_TtR = sqrt( ((-f_VehHalfWidth - f_TarY)*(-f_VehHalfWidth - f_TarY)) + ((f_TarX - f_xHFR)*(f_TarX - f_xHFR)) ) / (f_TarVelr);
    f_TtL = sqrt( ((f_VehHalfWidth - f_TarY)*(f_VehHalfWidth - f_TarY)) + ((f_TarX - f_xHFL - dxDiffObjCoord2VehCoord)*(f_TarX - f_xHFL - dxDiffObjCoord2VehCoord)) ) / (f_TarVelr);
    f_TtR = sqrt( ((-f_VehHalfWidth - f_TarY)*(-f_VehHalfWidth - f_TarY)) + ((f_TarX - f_xHFR - dxDiffObjCoord2VehCoord)*(f_TarX - f_xHFR - dxDiffObjCoord2VehCoord)) ) / (f_TarVelr);
    
    if (f_TtL > f_TtR)
       SideOfTar = 3; %% Target position, inLane 1, left 2, right 3
       f_tTRStart = f_TtR;
       f_tTLEnd = f_TtL;
    else
       SideOfTar = 2;
       f_tTLStart = f_TtL;
       f_tTREnd = f_TtR;
    end
    
    if (abs(f_HostVrel) < EPSILON)
        f_HostVrel = EPSILON;
    end
    
    %% host front reach the crossing left/right points
    f_TCHFLinearL = f_xHFL / f_HostVrel;
    f_TCHFLinearR = f_xHFR / f_HostVrel;
    
    %% host rear reach the crossing left/right points
    f_TCHRLinearL = f_TCHFLinearL + (f_VehLength / f_HostVrel);
    f_TCHRLinearR = f_TCHFLinearR + (f_VehLength / f_HostVrel);
end

== matlab function ObjSelect_lib/CD_CalculateTTI_CT_LinearPointMid/CD_CalculateTTI_CT_LinearPointMid ==
  data: VehHalfWidth input; f_TTCsec output; dxObj_Trans input; dyObj_Trans input; vxObj_Trans input; vyObj_Trans input; EPSILON input; VehSpdMps input; u_CollisionWay output; dxDiffObjCoord2VehCoord input
function [f_TTCsec,u_CollisionWay] = fcn(VehHalfWidth,dxObj_Trans,dyObj_Trans,vxObj_Trans,vyObj_Trans,EPSILON,VehSpdMps,dxDiffObjCoord2VehCoord)

f_VehHalfWidth = VehHalfWidth;
f_TarX = dxObj_Trans;
f_TarY = dyObj_Trans;
f_TarVelX = vxObj_Trans;
f_TarVelY = vyObj_Trans;
f_HostVrel = VehSpdMps;

f_VrelativeX = f_HostVrel - f_TarVelX;
f_RrelativeX = f_TarX;

if (f_VrelativeX < -0.001)
    %% no collision expected -> TTI to DEFAULT
    %f_TTLe = 25.5;
    %f_TTRi = 25.5;
    f_TTCsec = single(25.5);
    u_CollisionWay = uint8(0); %% no collision
else
    if ( abs(f_VrelativeX) > EPSILON )
        f_VXslop = 1/(abs(f_VrelativeX));
    else
        f_VXslop = single(1000.0);
    end

    %%f_Tt = f_RrelativeX *f_VXslop;
    f_Tt = (f_RrelativeX - dxDiffObjCoord2VehCoord) *f_VXslop;
    f_yHF = f_TarY + (f_Tt * f_TarVelY);
    
    if ( (f_yHF > -f_VehHalfWidth) && (f_yHF < f_VehHalfWidth) )
        f_TTCsec = f_Tt;
        u_CollisionWay = uint8(100); %% hit in lane
    elseif ( f_yHF > f_VehHalfWidth )
        f_TTCsec = single(25.5);
        u_CollisionWay = uint8(101); %% off the left side
    else
        f_TTCsec = single(25.5);
        u_CollisionWay = uint8(102); %% off the right side
    end
end
